simulink model "ACC_Sample"  (R2025a)
settings: Solver=VariableStepAuto  StartTime=0.0  StopTime=ell*T  RelTol=1e-3
values from neighbouring files (symbols this model uses):
  M = 2000    [ACC_data.mat]    (also in LK_data.mat = 1650)
  T = 0.2    [ACC_data.mat]    (also in LK_data.mat = 0.1)
  vkv = 0.2    [ACC_data.mat]
  vkx = 0.5    [ACC_data.mat]
  x0 = [79.6587016222 17.5244144376]    [ACC_data.mat]
libraries: autolibshared x1
settings Model: Creator=12775  LastModifiedBy=12775

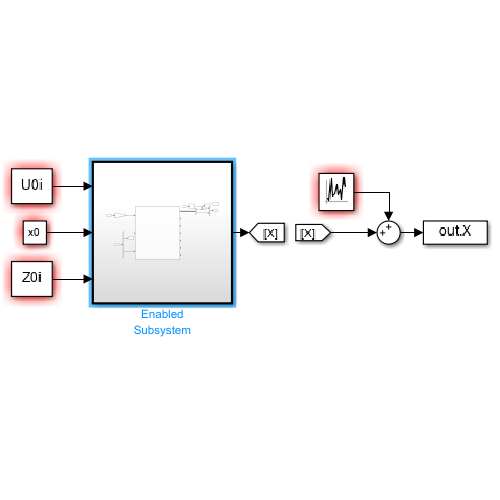
[thumbnail: Simulink's stored preview of the top-level diagram]
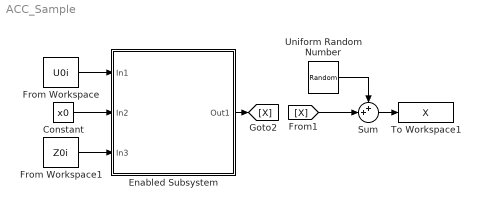
== system ACC_Sample ==
  Constant : Constant  Value=x0
  Enabled Subsystem : Subsystem  TreatAsAtomicUnit=on
  From Workspace : FromWorkspace  VariableName=U0i  SampleTime=T
  From Workspace1 : FromWorkspace  VariableName=Z0i  SampleTime=T
  Sum : Sum  Inputs=++|
  To Workspace1 : ToWorkspace  VariableName=X  SampleTime=T
  Uniform Random Number : UniformRandomNumber  Minimum=[-vkx;-vkv]  Maximum=[vkx;vkv]  Seed=[1,2]  SampleTime=T
  wires:
  Enabled Subsystem/1(Out1) -> [X]
  From Workspace1/1 -> Enabled Subsystem/3(In3)
  Constant/1 -> Enabled Subsystem/2(In2)
  From Workspace/1 -> Enabled Subsystem/1(In1)
  Sum/1 -> To Workspace1/1
  [X] -> Sum/2
  Uniform Random Number/1 -> Sum/1

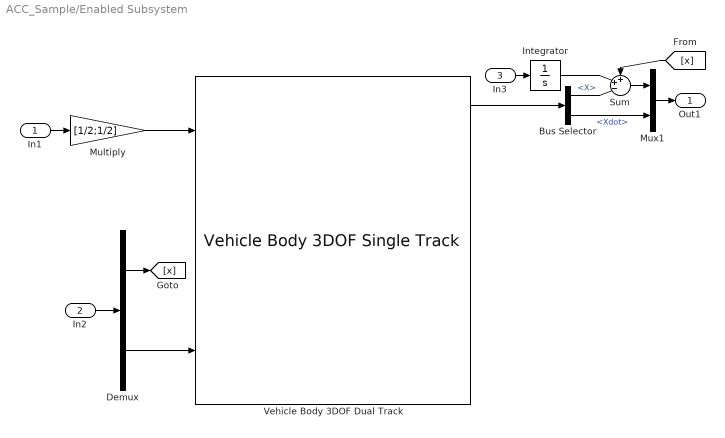
== system ACC_Sample/Enabled Subsystem ==
  In1 : Inport
  In2 : Inport  Port=2
  In3 : Inport  Port=3
  Bus Selector : BusSelector  OutputSignals=InertFrm.Cg.Disp.X,InertFrm.Cg.Vel.Xdot
  Demux : Demux  Outputs=2
  Integrator : Integrator
  Multiply : Gain  Gain=[1/2;1/2]
  Mux1 : Mux  Inputs=2
  Sum : Sum  Inputs=++-|
  Vehicle Body 3DOF Dual Track : autolibshared/Vehicle Body 3DOF Single Track  trackMode=Dual  inputMode=External longitudinal forces  frontSteerMode=off  rearSteerMode=off  windMode=off  muMode=off  extFMode=off  extMMode=off  htchFMode=off  htchMMode=off  extXo=off  extpsio=off  extxdoto=on  extro=off  extYo=off  extTamb=off  extydoto=off  aMode=2  NF=2  NR=2  m=M  a=1.4  b=1.6  h=0.35  dh=1  hh=0.2  X_o=0  xdot_o=0  CalphaMode=off  sigmaMode=on  d=0  hl=0  w=[1.4,1.4]  Cy_f=12e3  Cy_r=11e3  sigma_f=.1  sigma_r=.1  alpha_f_brk=[-.1 .1]  Cy_f_data=[-9e3 9e3]  alpha_r_brk=[-.1 .1]  Cy_r_data=[-9e3 9e3]  Y_o=0  ydot_o=0  Izz=4000  psi_o=0  r_o=0  Af=2  Cd=.3  Cl=.1  Cpm=.1  beta_w=[0 0.01:0.01:0.3]  Cs=[0:0.03:0.9]  Cym=[0 1e-6:0.01:0.3]  Pabs=101325  Tair=273  g=9.81  mu=1  xdot_tol=.01  Fznom=5000  Fxtire_sat=7e4  Fytire_sat=7e4  longOff=0  latOff=0  vertOff=0  wrapAng=off
      settings: LibrarySourceBlock=vehdynlibeom/Vehicle Body 3DOF Dual Track
  Out1 : Outport
  wires:
  In2/1 -> Demux/1
  Sum/1 -> Mux1/1
  Demux/1 -> [x]
  In3/1 -> Integrator/1
  Bus Selector/1 -> Sum/3  "<X>"
  [x] -> Sum/1
  Vehicle Body 3DOF Dual Track/1 -> Bus Selector/1
  Multiply/1 -> Vehicle Body 3DOF Dual Track/1
  Integrator/1 -> Sum/2
  Mux1/1 -> Out1/1
  Bus Selector/2 -> Mux1/2  "<Xdot>"
  Demux/2 -> Vehicle Body 3DOF Dual Track/3
  In1/1 -> Multiply/1
